simulink library "cooperative"  (Simulink 7.4)
settings: Solver=ode45  SolverMode=SingleTasking  StartTime=0.0  StopTime=10.0  RelTol=1e-3
undefined symbols (not defined in the file): ATRFunctions, g_AssignmentAlgorithm, g_CommandTurnRadius, g_CoordinationDelayDen, g_DefaultWaypointAltitude, g_EntityTypes, g_MaxNumberTargets, g_MaxNumberVehicles, g_MaxReassignmentDeltaTime, g_ObjectMessageIDs, g_OptionSaveDataAVDS, g_SampleTime, g_SensorRollLimitDeg, g_TargetStates, g_Tasks, g_TruthMemory, g_TypeAssignment, g_VehicleInputFiles, g_VehicleMemory, g_VehicleTypes, g_WaypointDefinitions, g_WaypointTypes
libraries: cooperative x23
(part 3 of 3)

== system cooperative/UAV1/ReceiveTruth/ImplementNewAssignment/VehicleAlive ==
  In1 : Inport
  In2 : Inport  Port=2
  Enable : EnablePort
  Bus Selector1 : BusSelector  OutputSignals=ChangeAssignmentFlagSelf
  Greater : Subsystem
  NewAssignment : Subsystem  TreatAsAtomicUnit=on
  Selector : Selector  InputPortWidth=g_MaxNumberVehicles  IndexOptions=Index vector (port)  Indices=[1 3]  OutputSizes=1
  wires:
  Bus Selector1/1 -> Selector/1  "<ChangeAssignmentFlagSelf>"
  Selector/1 -> Greater/1(Signal)
  In1/1 -> NewAssignment/1(VehicleID), Selector/2
  Greater/1(Greater?) -> NewAssignment/Enable
  In2/1 -> Bus Selector1/1

== system cooperative/UAV1/SendMessages/SendATRTime/Enabled Subsystem ==
  ATRTime : Inport
  Enable : EnablePort
  Digital Clock : DigitalClock  SampleTime=g_SampleTime
  SaveWaypointIndex : DataStoreWrite  DataStoreName=ATRTime  SampleTime=g_SampleTime
  TimeStamp : Outport
  wires:
  ATRTime/1 -> SaveWaypointIndex/1
  Digital Clock/1 -> TimeStamp/1

== system cooperative/UAV1/SendMessages/SendAuctionData/Enabled Subsystem ==
  MessageNumber : Inport
  Enable : EnablePort
  Data Store Write : DataStoreWrite  DataStoreName=LastMessageNumber  SampleTime=g_SampleTime
  Digital Clock : DigitalClock  SampleTime=g_SampleTime
  TimeStamp : Outport
  wires:
  MessageNumber/1 -> Data Store Write/1
  Digital Clock/1 -> TimeStamp/1

== system cooperative/UAV1/SendMessages/SendChangedStatus/Enabled Subsystem ==
  Enable : EnablePort
  Digital Clock : DigitalClock  SampleTime=g_SampleTime
  TimeStamp : Outport
  wires:
  Digital Clock/1 -> TimeStamp/1

== system cooperative/UAV1/SendMessages/SendPositionFlag/Enabled Subsystem ==
  PositionFlag : Inport
  Enable : EnablePort
  Digital Clock : DigitalClock  SampleTime=g_SampleTime
  SaveWaypointIndex : DataStoreWrite  DataStoreName=PositionFlag  SampleTime=g_SampleTime
  TimeStamp : Outport
  wires:
  Digital Clock/1 -> TimeStamp/1
  PositionFlag/1 -> SaveWaypointIndex/1

== system cooperative/UAV1/SendMessages/SendPositionID/Enabled Subsystem ==
  PositionSendFlag Time : Inport
  Enable : EnablePort
  Data Store Write : DataStoreWrite  DataStoreName=PositionsSendFlagTime  SampleTime=g_SampleTime
  Digital Clock : DigitalClock  SampleTime=g_SampleTime
  TimeStamp : Outport
  wires:
  PositionSendFlag Time/1 -> Data Store Write/1
  Digital Clock/1 -> TimeStamp/1

== system cooperative/UAV1/SendMessages/SendTargetAttacked/Enabled Subsystem ==
  "TargetAttacked " : Inport
  Enable : EnablePort
  Digital Clock : DigitalClock  SampleTime=g_SampleTime
  SaveWaypointIndex : DataStoreWrite  DataStoreName=TargetAttacked  SampleTime=g_SampleTime
  TimeStamp : Outport
  wires:
  Digital Clock/1 -> TimeStamp/1
  "TargetAttacked "/1 -> SaveWaypointIndex/1

== system cooperative/UAV1/SendMessages/SendTargetStatus/Enabled Subsystem ==
  Enable : EnablePort
  Digital Clock : DigitalClock  SampleTime=g_SampleTime
  TimeStamp : Outport
  wires:
  Digital Clock/1 -> TimeStamp/1

== system cooperative/UAV1/SendMessages/SendTaskBenefits/Enabled Subsystem ==
  ReplanRound : Inport
  Enable : EnablePort
  Data Store Write : DataStoreWrite  DataStoreName=LastReplanRound  SampleTime=g_SampleTime
  Digital Clock : DigitalClock  SampleTime=g_SampleTime
  TimeStamp : Outport
  wires:
  ReplanRound/1 -> Data Store Write/1
  Digital Clock/1 -> TimeStamp/1

== system cooperative/UAV1/SendMessages/SendTriggerReplan/Enabled Subsystem ==
  Enable : EnablePort
  Digital Clock : DigitalClock  SampleTime=g_SampleTime
  TimeStamp : Outport
  wires:
  Digital Clock/1 -> TimeStamp/1

== system cooperative/UAV1/SendMessages/SendWaypointNumber/Enabled Subsystem ==
  Waypoint : Inport
  Enable : EnablePort
  Digital Clock : DigitalClock  SampleTime=g_SampleTime
  SaveWaypointIndex : DataStoreWrite  DataStoreName=WaypoinNumber  SampleTime=g_SampleTime
  TimeStamp : Outport
  wires:
  Digital Clock/1 -> TimeStamp/1
  Waypoint/1 -> SaveWaypointIndex/1

== system cooperative/UAV1/SendTruth/SendNewAssignment/Changed1 ==
  Signal : Inport
  Relational Operator3 : RelationalOperator  Operator=>  InputSameDT=on
  Unit Delay : UnitDelay  SampleTime=g_SampleTime
  Greater? : Outport
  wires:
  Unit Delay/1 -> Relational Operator3/2
  Relational Operator3/1 -> Greater?/1
  Signal/1 -> Relational Operator3/1, Unit Delay/1

== system cooperative/UAV1/SendTruth/SendNewAssignment/Enabled Subsystem ==
  Enable : EnablePort
  Digital Clock : DigitalClock  SampleTime=g_SampleTime
  TimeStamp : Outport
  wires:
  Digital Clock/1 -> TimeStamp/1

== system cooperative/UAV1/SendTruth/SendTargetStatus/Enabled Subsystem ==
  TargetStatus : Inport
  Enable : EnablePort
  Data Store Write : DataStoreWrite  DataStoreName=TargetStatus  SampleTime=g_SampleTime
  Digital Clock : DigitalClock  SampleTime=g_SampleTime
  TimeStamp : Outport
  wires:
  Digital Clock/1 -> TimeStamp/1
  TargetStatus/1 -> Data Store Write/1

== system cooperative/UAV1/SendTruth/SendTrackList/Enabled Subsystem ==
  TrackList : Inport
  Enable : EnablePort
  Data Store Write : DataStoreWrite  DataStoreName=TrackList  SampleTime=g_SampleTime
  Digital Clock : DigitalClock  SampleTime=g_SampleTime
  TimeStamp : Outport
  wires:
  Digital Clock/1 -> TimeStamp/1
  TrackList/1 -> Data Store Write/1

== system cooperative/UAV1/SendTruth/SendVehicleIsDead/Enabled Subsystem ==
  State : Inport
  Enable : EnablePort
  Digital Clock : DigitalClock  SampleTime=g_SampleTime
  Save : DataStoreWrite  DataStoreName=VehicleIDead  SampleTime=g_SampleTime
  TimeStamp : Outport
  wires:
  Digital Clock/1 -> TimeStamp/1
  State/1 -> Save/1

== system cooperative/UAV1/SendTruth/SendWeaponsRelease/Enabled Subsystem ==
  WeaponID : Inport
  Enable : EnablePort
  Data Store Write : DataStoreWrite  DataStoreName=WeaponID  SampleTime=g_SampleTime
  Digital Clock : DigitalClock  SampleTime=g_SampleTime
  TimeStamp : Outport
  wires:
  WeaponID/1 -> Data Store Write/1
  Digital Clock/1 -> TimeStamp/1

== system cooperative/UAV1/EmbeddedFlightSoftware/CooperationManager/Calculate Assignment/CapTransShip ==
  note: Calculate Assignment
      |
      | PURPOSE: Calculate the assignments for the vehicles based on the current
      |      state of the targets and vehicles.
      |
      | IMPLEMENTATION:
      | - CapTransShipIO - calculates the costs/bennefits associated with the vehicle
      |      task assignments. "CapTransShipIO" also formats the data into the input
      |      form expected by the assignment algorithm.
      | - Capacitative Transshipment Solver - this is an interface to a compiled S-function
      |      that implements a capacitated transhipment algorithm. It is used to select the
      |      target and task assignment for all of the vehicles.
      | - Assignment for Local Vehicle - uses the current vehicle's ID to select and output
      |      the target and task assignment for this vehicle.
  ComBusLocalIn : Inport  SampleTime=g_SampleTime
  ComBusIn : Inport  Port=2  SampleTime=g_SampleTime
  Enable : EnablePort
  Assignment for Local Vehicle : Subsystem
  Bus Selector1 : BusSelector  OutputSignals=VehicleID,EFS(com).TargetManager(com).Target Status.TargetStatus  OutputAsBus=on
  Bus Selector2 : BusSelector  OutputSignals=ETACostToSearch,TargetAttacked  OutputAsBus=on
  CapTransShipIOInS : S-Function  FunctionName=CapTransShipIOInS  Parameters=g_MaxNumberTargets,g_MaxNumberVehicles,g_Tasks.NumberTasks  EnableBusSupport=off
  Capacitative Transshipment Solver : S-Function  FunctionName=CapTranShipDll  Parameters=g_MaxNumberVehicles,g_MaxNumberTargets,g_Tasks.NumberTasks  EnableBusSupport=off
  Mux3 : Mux  Inputs=2
  Local Assignment : Outport  InitialOutput=[0,0,0]
  wires:
  Assignment for Local Vehicle/1(Out1) -> Local Assignment/1
  ComBusIn/1 -> Bus Selector2/1
  CapTransShipIOInS/1 -> Capacitative Transshipment Solver/1
  Mux3/1 -> CapTransShipIOInS/1
  Capacitative Transshipment Solver/1 -> Assignment for Local Vehicle/2(In2)  "Assignment"
  Bus Selector1/1 -> Mux3/1
  ComBusLocalIn/1 -> Bus Selector1/1, Assignment for Local Vehicle/1(In1)
  Bus Selector2/1 -> Mux3/2

== system cooperative/UAV1/EmbeddedFlightSoftware/CooperationManager/Calculate Assignment/DistAuctItCapTransShip ==
  ComBusLocalIn : Inport  SampleTime=g_SampleTime
  ComBusIn : Inport  Port=2  SampleTime=g_SampleTime
  SimBusIn : Inport  Port=3  SampleTime=g_SampleTime
  EnableType : Inport  Port=4  SampleTime=g_SampleTime
  Enable : EnablePort
  Assignment Algorithm : Subsystem
  Bus Creator : BusCreator  Inputs=2
  Message Processing : Subsystem
  Not Used : Constant  Value=[0 0]
  Replan Logic : Subsystem
  Store Benefits : Subsystem  TreatAsAtomicUnit=on
  Local Assignment : Outport
  AuctionData : Outport  Port=2
  wires:
  EnableType/1 -> Replan Logic/1(EnableType)
  Store Benefits/1(BenefitsStored) -> Assignment Algorithm/3(StoredBenefits)
  Assignment Algorithm/2(TargetStates) -> Store Benefits/3(TargetStates)
  Assignment Algorithm/3(StoreBenefits) -> Store Benefits/Enable
  Message Processing/1(NewBid) -> Assignment Algorithm/1(NewBid)
  Message Processing/2(NewAssignment) -> Assignment Algorithm/2(NewAssignment)
  Message Processing/3(RoundComplete) -> Assignment Algorithm/4(RoundComplete)
  Assignment Algorithm/1(AuctionData) -> AuctionData/1  "AuctionData"
  Replan Logic/1(ReplanTrigger) -> Assignment Algorithm/5(ReplanTrigger), Message Processing/4(ReplanTrigger)  "ReplanTrigger"
  ComBusLocalIn/1 -> Assignment Algorithm/6(CommBusLocalIn), Store Benefits/2(CommBusLocalIn), Message Processing/3(CommBusLocalIn)
  SimBusIn/1 -> Message Processing/2(SimBusIn)
  ComBusIn/1 -> Store Benefits/1(CommBusIn), Message Processing/1(CommBusIn)
  Not Used/1 -> Bus Creator/1
  Bus Creator/1 -> Local Assignment/1
  Assignment Algorithm/4(NewAssignmentTime) -> Bus Creator/2  "NewAssignmetTime"

== system cooperative/UAV1/EmbeddedFlightSoftware/CooperationManager/Calculate Assignment/DistItCapTransShip ==
  ComBusLocalIn : Inport  SampleTime=g_SampleTime
  ComBusIn : Inport  Port=2  SampleTime=g_SampleTime
  SimBusIn : Inport  Port=3  SampleTime=g_SampleTime
  EnableType : Inport  Port=4  SampleTime=g_SampleTime
  Enable : EnablePort
  Assignment Algorithm : Subsystem
  Bus Creator : BusCreator  Inputs=2
  Demux : Demux  Outputs=7  BusSelectionMode=on
  Iteration Logic : Subsystem
  Mux : Mux  Inputs=7
  Not Used : Constant  Value=[0 0]
  Replan Logic : Subsystem
  Send Benefits : Subsystem  TreatAsAtomicUnit=on
  Local Assignment : Outport  InitialOutput=[0,0,0]
  Algorithm Data : Outport  Port=2
  wires:
  EnableType/1 -> Replan Logic/1(EnableType)
  Assignment Algorithm/3(SendBenefitsTrigger) -> Send Benefits/Enable
  Assignment Algorithm/1(TargetStatesOut) -> Send Benefits/3(TargetStates)
  Assignment Algorithm/2(ReplanRoundOut) -> Send Benefits/4(ReplanRound)
  Replan Logic/1(ReplanTrigger) -> Assignment Algorithm/8(ReplanTrigger)
  Demux/7 -> Assignment Algorithm/7(Sync)
  Demux/6 -> Assignment Algorithm/6(SearchBenefits)
  Demux/5 -> Assignment Algorithm/5(TimeToComplete)
  Demux/4 -> Assignment Algorithm/4(TaskBenefits)
  Demux/3 -> Assignment Algorithm/3(TargetStatesIn)
  Demux/2 -> Assignment Algorithm/2(ReplanRoundIn)
  Demux/1 -> Assignment Algorithm/1(ActiveVehicles)
  Mux/1 -> Demux/1
  Iteration Logic/7(Sync) -> Mux/7
  Iteration Logic/6(SearchBenefits) -> Mux/6
  Iteration Logic/5(TimeToComplete) -> Mux/5
  Iteration Logic/4(TaskBenefits) -> Mux/4
  Iteration Logic/3(TargetStates) -> Mux/3
  Iteration Logic/2(ReplanRound) -> Mux/2
  Iteration Logic/1(ActiveVehicles) -> Mux/1
  ComBusLocalIn/1 -> Assignment Algorithm/9(CommBusLocalIn), Send Benefits/2(CommBusLocalIn)
  SimBusIn/1 -> Iteration Logic/2(SimBusIn)
  ComBusIn/1 -> Send Benefits/1(CommBusIn), Iteration Logic/1(CommBusIn)
  Send Benefits/1(Algorithm Data) -> Algorithm Data/1
  Not Used/1 -> Bus Creator/1  "Localassignment"
  Bus Creator/1 -> Local Assignment/1
  Assignment Algorithm/4(NewAssignmentTime) -> Bus Creator/2  "NewAssignmentTime"

== system cooperative/UAV1/EmbeddedFlightSoftware/CooperationManager/Calculate Assignment/ItCapTransShip ==
  note: ItCapTransShip
      |
      | PURPOSE: .
      |
      | IMPLEMENTATION:
      | - .
      | - .
      | - .
  ComBusLocalIn : Inport  SampleTime=g_SampleTime
  ComBusIn : Inport  Port=2  SampleTime=g_SampleTime
  SimBusIn : Inport  Port=3  SampleTime=g_SampleTime
  Enable : EnablePort
  Bus Selector : BusSelector  OutputSignals=PositionID,WaypointIndex,TriggerReplan  OutputAsBus=on
  Bus Selector1 : BusSelector  OutputSignals=VehicleID,EFS(com).TargetManager(com).SensedTargetInformation.Targets,EFS(com).TargetManager(com).Target Status.TargetStatus,EFS(com).SensorManager(com).ATR Combined.Desired Headings.DesiredHeadings01,EFS(com).SensorManager(com).ATR Combined.Desired Headings.DesiredHeadings02,EFS(com).SensorManager(com).ATR Combined.Desired Headings.DesiredHeadings03,EFS(com).SensorManager(com).ATR Combined.Desired Headings.DesiredHeadings04,Dynamics(com).TacticalManuevering.CommandTurnRadius,Dynamics(com).TacticalManuevering.WayPointNumber,Dynamics(com).TacticalManuevering.WayPointTypeCurrent  OutputAsBus=on
  Bus Selector2 : BusSelector  OutputSignals=ExternalTruth.VehicleIsDead  OutputAsBus=on
  MultiTaskAssignIOS : S-Function  FunctionName=MultiTaskAssignIOS  Parameters=g_TypeAssignment.ItCapTransShip,g_MaxNumberTargets,g_MaxNumberVehicles  EnableBusSupport=off
  Mux : Mux  Inputs=3
  Local Assignment : Outport  InitialOutput=[0,0,0]
  wires:
  Bus Selector2/1 -> Mux/2
  SimBusIn/1 -> Bus Selector2/1
  Mux/1 -> MultiTaskAssignIOS/1
  Bus Selector1/1 -> Mux/3
  Bus Selector/1 -> Mux/1
  MultiTaskAssignIOS/1 -> Local Assignment/1
  ComBusIn/1 -> Bus Selector/1
  ComBusLocalIn/1 -> Bus Selector1/1

== system cooperative/UAV1/EmbeddedFlightSoftware/CooperationManager/Calculate Assignment/ItJacobi ==
  note: ItCapTransShip
      |
      | PURPOSE: .
      |
      | IMPLEMENTATION:
      | - .
      | - .
      | - .
  ComBusLocalIn : Inport  SampleTime=g_SampleTime
  ComBusIn : Inport  Port=2  SampleTime=g_SampleTime
  SimBusIn : Inport  Port=3  SampleTime=g_SampleTime
  Enable : EnablePort
  Bus Selector : BusSelector  OutputSignals=PositionID,WaypointIndex,TriggerReplan  OutputAsBus=on
  Bus Selector1 : BusSelector  OutputSignals=VehicleID,EFS(com).TargetManager(com).SensedTargetInformation.Targets,EFS(com).TargetManager(com).Target Status.TargetStatus,EFS(com).SensorManager(com).ATR Combined.Desired Headings.DesiredHeadings01,EFS(com).SensorManager(com).ATR Combined.Desired Headings.DesiredHeadings02,EFS(com).SensorManager(com).ATR Combined.Desired Headings.DesiredHeadings03,EFS(com).SensorManager(com).ATR Combined.Desired Headings.DesiredHeadings04,Dynamics(com).TacticalManuevering.CommandTurnRadius,Dynamics(com).TacticalManuevering.WayPointNumber,Dynamics(com).TacticalManuevering.WayPointTypeCurrent  OutputAsBus=on
  Bus Selector3 : BusSelector  OutputSignals=ExternalTruth.VehicleIsDead  OutputAsBus=on
  MultiTaskAssignIOS : S-Function  FunctionName=MultiTaskAssignIOS  Parameters=g_TypeAssignment.ItAuctionJacobi,g_MaxNumberTargets,g_MaxNumberVehicles  EnableBusSupport=off
  Mux : Mux  Inputs=3
  Local Assignment : Outport  InitialOutput=[0,0,0]
  wires:
  Bus Selector3/1 -> Mux/2
  SimBusIn/1 -> Bus Selector3/1
  Mux/1 -> MultiTaskAssignIOS/1
  Bus Selector1/1 -> Mux/3
  Bus Selector/1 -> Mux/1
  MultiTaskAssignIOS/1 -> Local Assignment/1
  ComBusIn/1 -> Bus Selector/1
  ComBusLocalIn/1 -> Bus Selector1/1

== system cooperative/UAV1/EmbeddedFlightSoftware/CooperationManager/Calculate Assignment/MessageDisplay ==
  In1 : Inport
  Enable : EnablePort
  MessageDisplayS : S-Function  Priority=1  FunctionName=MessageDisplayS  Parameters='Replan'  EnableBusSupport=off
  wires:
  In1/1 -> MessageDisplayS/1

== system cooperative/UAV1/EmbeddedFlightSoftware/CooperationManager/Calculate Assignment/Relative Bennifits ==
  note: ItCapTransShip
      |
      | PURPOSE: .
      |
      | IMPLEMENTATION:
      | - .
      | - .
      | - .
  ComBusLocalIn : Inport  SampleTime=g_SampleTime
  ComBusIn : Inport  Port=2  SampleTime=g_SampleTime
  SimBusIn : Inport  Port=3  SampleTime=g_SampleTime
  Enable : EnablePort
  Bus Selector1 : BusSelector  OutputSignals=VehicleID,EFS(com).TargetManager(com).SensedTargetInformation.Targets,EFS(com).TargetManager(com).Target Status.TargetStatus,EFS(com).SensorManager(com).ATR Combined.Desired Headings.DesiredHeadings01,EFS(com).SensorManager(com).ATR Combined.Desired Headings.DesiredHeadings02,EFS(com).SensorManager(com).ATR Combined.Desired Headings.DesiredHeadings03,EFS(com).SensorManager(com).ATR Combined.Desired Headings.DesiredHeadings04,Dynamics(com).TacticalManuevering.CommandTurnRadius,Dynamics(com).TacticalManuevering.WayPointNumber,Dynamics(com).TacticalManuevering.WayPointTypeCurrent  OutputAsBus=on
  Bus Selector3 : BusSelector  OutputSignals=PositionID,WaypointIndex,TriggerReplan  OutputAsBus=on
  Bus Selector4 : BusSelector  OutputSignals=ExternalTruth.VehicleIsDead  OutputAsBus=on
  MultiTaskAssignIOS : S-Function  FunctionName=MultiTaskAssignIOS  Parameters=g_TypeAssignment.RelativeBenefits,g_MaxNumberTargets,g_MaxNumberVehicles  EnableBusSupport=off
  Mux : Mux  Inputs=3
  Local Assignment : Outport  InitialOutput=[0,0,0]
  wires:
  Bus Selector4/1 -> Mux/2
  SimBusIn/1 -> Bus Selector4/1
  Mux/1 -> MultiTaskAssignIOS/1
  Bus Selector1/1 -> Mux/3
  Bus Selector3/1 -> Mux/1
  MultiTaskAssignIOS/1 -> Local Assignment/1
  ComBusIn/1 -> Bus Selector3/1
  ComBusLocalIn/1 -> Bus Selector1/1

== system cooperative/UAV1/EmbeddedFlightSoftware/CooperationManager/Enable Reassignment/Assignment Time Delay ==
  note: Coordination Timing
      |
      | PURPOSE: This is a time delay to make sure that all of the
      |  other vehicle have had time to calculate the new
      |  routes. If they still have not the replan algorithm will
      |  not use that vehicle's old information.
  In : Inport  SampleTime=g_SampleTime
  Discrete Transfer Fcn : DiscreteTransferFcn  Denominator=g_CoordinationDelayDen  SampleTime=g_SampleTime
  InDelayed : Outport
  wires:
  Discrete Transfer Fcn/1 -> InDelayed/1
  In/1 -> Discrete Transfer Fcn/1

== system cooperative/UAV1/EmbeddedFlightSoftware/CooperationManager/Enable Reassignment/Changed ==
  Signal : Inport
  Relational Operator3 : RelationalOperator  Operator=~=  InputSameDT=on
  Unit Delay : UnitDelay  SampleTime=g_SampleTime
  Increased? : Outport
  wires:
  Unit Delay/1 -> Relational Operator3/2
  Relational Operator3/1 -> Increased?/1
  Signal/1 -> Relational Operator3/1, Unit Delay/1

== system cooperative/UAV1/EmbeddedFlightSoftware/CooperationManager/Enable Reassignment/Changed1 ==
  Signal : Inport
  Relational Operator3 : RelationalOperator  Operator=~=  InputSameDT=on
  Unit Delay : UnitDelay  SampleTime=g_SampleTime
  Changed? : Outport
  wires:
  Unit Delay/1 -> Relational Operator3/2
  Relational Operator3/1 -> Changed?/1
  Signal/1 -> Relational Operator3/1, Unit Delay/1

== system cooperative/UAV1/EmbeddedFlightSoftware/CooperationManager/Enable Reassignment/Changed2 ==
  Signal : Inport
  Relational Operator3 : RelationalOperator  Operator=~=  InputSameDT=on
  Unit Delay : UnitDelay  SampleTime=g_SampleTime
  Changed? : Outport
  wires:
  Signal/1 -> Unit Delay/1, Relational Operator3/1
  Relational Operator3/1 -> Changed?/1
  Unit Delay/1 -> Relational Operator3/2

== system cooperative/UAV1/EmbeddedFlightSoftware/CooperationManager/Task List/Update Task List ==
  note: Task List
  Vehicle ID : Inport  SampleTime=g_SampleTime
  TargetStatus : Inport  Port=2  SampleTime=g_SampleTime
  Enable : EnablePort
  Mux : Mux  Inputs=2
  TargetStatusS : S-Function  FunctionName=TaskListS  Parameters=g_MaxNumberTargets  EnableBusSupport=off
  "Write Last Target Status " : DataStoreWrite  DataStoreName=LastTargetStatus  SampleTime=g_SampleTime
  UnassignedTaskFlag : Outport
  wires:
  TargetStatusS/1 -> UnassignedTaskFlag/1
  Mux/1 -> TargetStatusS/1
  Vehicle ID/1 -> Mux/1
  TargetStatus/1 -> Mux/2, "Write Last Target Status "/1

== system cooperative/UAV1/EmbeddedFlightSoftware/RouteManager/ReplanSingle/Replan ==
  note: RouteSelection
      |
      | PURPOSE: Calculates the ETA, cost and waypoint trajectory for the lowest
      |      cost flyable path to each of the targets, to accomplish the appropriate task,
      |      and stores the data for later use.
      |
      | Implementation:
      | - ReplanRoutes- calls the function, "ReplanRoutes" to do the calculations. The
      |      lowest cost set of waypoints for each known target is stored in the appropriate
      |      location in the global structure "VehicleMemory.RouteManager".
  In1 : Inport
  Enable : EnablePort
  Bus Creator : BusCreator
  Bus Selector : BusSelector  OutputSignals=Local Bus.VehicleID,Vehicle (Sim).EFS(sim).RouteManager(sim).VehicleFinished.Vehicle Finished,Local Bus.Dynamics(com).TacticalManuevering.CommandTurnRadius,Local Bus.Dynamics(com).AC Dynamics.Position_x,Local Bus.Dynamics(com).AC Dynamics.Position_y,Local Bus.Dynamics(com).AC Dynamics.Altitude,Local Bus.Dynamics(com).AC Dynamics.Psi,Local Bus.Dynamics(com).AC Dynamics.V North,Local Bus.Dynamics(com).AC Dynamics.V East,Local Bus.Dynamics(com).TacticalManuevering.CommandVelocity,Local Bus.Dynamics(com).TacticalManuevering.WayPointNumber,Local Bus.EFS(com).RouteManager(com).TaskStatus.Task Finished,Local Bus.EFS(com).TargetManager(com).Target Status.TargetStatus,Local Bus.EFS(com).SensorManager(com).ATR Combined.Desired Headings,TargetState  OutputAsBus=on
  Demux : Demux  Outputs=[g_MaxNumberTargets,g_MaxNumberTargets,g_MaxNumberTargets]
  Digital Clock : DigitalClock  SampleTime=g_SampleTime
  ReplanRoutes : S-Function  FunctionName=ReplanRoutesS  Parameters=g_MaxNumberTargets  EnableBusSupport=off
  ReplanETAsCosts : Outport
  wires:
  Demux/2 -> Bus Creator/3  "TargetETAs"
  Digital Clock/1 -> Bus Creator/1  "ReplanTime"
  In1/1 -> Bus Selector/1
  Bus Selector/1 -> ReplanRoutes/1
  Demux/3 -> Bus Creator/4  "TargetToSearchDist"
  Bus Creator/1 -> ReplanETAsCosts/1  "Replan ETAs and Costs"
  ReplanRoutes/1 -> Demux/1
  Demux/1 -> Bus Creator/2  "TargetCosts"

== system cooperative/UAV1/EmbeddedFlightSoftware/RouteManager/ReplanSingle/RouteSelection ==
  note: RouteSelection
      |
      | PURPOSE: This manager implements waypoints for the route selected for this
      | vehicle during the vehicle/target assignment in the cooperation manager.
      |
      | Implementation:
      | - RouteSelection - calls the function "RouteSelection" to implement waypoints
      |      for the route selected.
  In1 : Inport
  Enable : EnablePort
  RouteSelection : S-Function  FunctionName=RouteSelectionS  EnableBusSupport=off
  wires:
  In1/1 -> RouteSelection/1

== system cooperative/UAV1/EmbeddedFlightSoftware/RouteManager/Task Status/Alive Time ==
  Local (Comm) : Inport  SampleTime=g_SampleTime
  Enable : EnablePort
  Bus Selector4 : BusSelector  OutputSignals=VehicleID
  Digital Clock : DigitalClock  SampleTime=g_SampleTime
  Mux : Mux  Inputs=2
  S-Function : S-Function  FunctionName=MonteCarloMetricS  Parameters='AliveTimeSeconds'  EnableBusSupport=off
  wires:
  Bus Selector4/1 -> Mux/1  "<VehicleID>"
  Local (Comm)/1 -> Bus Selector4/1
  Mux/1 -> S-Function/1
  Digital Clock/1 -> Mux/2

== system cooperative/UAV1/EmbeddedFlightSoftware/RouteManager/Task Status/D Latch ==
  Enable : Inport
  In : Inport  Port=2  SampleTime=g_SampleTime
  D Latch : Subsystem  TreatAsAtomicUnit=on
  Latched : Outport  InitialOutput=0
  wires:
  Enable/1 -> D Latch/Enable
  D Latch/1(Q) -> Latched/1
  In/1 -> D Latch/1(D)

== system cooperative/UAV1/EmbeddedFlightSoftware/RouteManager/Task Status/D Latch1 ==
  Enable : Inport
  In : Inport  Port=2  SampleTime=g_SampleTime
  D Latch : Subsystem  TreatAsAtomicUnit=on
  Latched : Outport  InitialOutput=0
  wires:
  In/1 -> D Latch/1(D)
  D Latch/1(Q) -> Latched/1
  Enable/1 -> D Latch/Enable

== system cooperative/UAV1/EmbeddedFlightSoftware/RouteManager/Task Status/D Latch2 ==
  Enable : Inport
  In : Inport  Port=2  SampleTime=g_SampleTime
  D Latch : Subsystem  TreatAsAtomicUnit=on
  Latched : Outport  InitialOutput=0
  wires:
  Enable/1 -> D Latch/Enable
  D Latch/1(Q) -> Latched/1
  In/1 -> D Latch/1(D)

== system cooperative/UAV1/EmbeddedFlightSoftware/RouteManager/Task Status/Task Failed Check ==
  Local (Comm) : Inport
  Bus Selector1 : BusSelector  OutputSignals=Dynamics(com).TacticalManuevering.WayPointTypeCurrent,EFS(com).TargetManager(com).Target Status.TargetStatus
  Create Last Task : DataStoreMemory  DataStoreName=LastWaypointType
  Create Last Task1 : DataStoreMemory  DataStoreName=LastTargetState  InitialValue=g_TargetStates.StateUndefined*ones(g_MaxNumberTargets,1)
  Logical Operator : Logic  Operator=OR
  Read Last Task : DataStoreRead  DataStoreName=LastWaypointType  SampleTime=g_SampleTime
  Read Last Task1 : DataStoreRead  DataStoreName=LastTargetState  SampleTime=g_SampleTime
  Relational Operator1 : RelationalOperator  Operator=~=  InputSameDT=on
  Relational Operator4 : RelationalOperator  Operator=~=  InputSameDT=on
  Task Failed Check : Subsystem  TreatAsAtomicUnit=on
  TaskFailed : Outport
  wires:
  Relational Operator1/1 -> Logical Operator/2
  Read Last Task1/1 -> Task Failed Check/2(LastTargetState), Relational Operator1/2
  Bus Selector1/2 -> Relational Operator1/1  "<TargetStatus>"
  Relational Operator4/1 -> Logical Operator/1
  Logical Operator/1 -> Task Failed Check/Enable
  Task Failed Check/1(TaskFailed) -> TaskFailed/1
  Bus Selector1/1 -> Relational Operator4/2  "<WayPointTypeCurrent>"
  Read Last Task/1 -> Relational Operator4/1
  Local (Comm)/1 -> Task Failed Check/1(Local (Comm)), Bus Selector1/1

== system cooperative/UAV1/EmbeddedFlightSoftware/RouteManager/Task Status/VehicleType ==
  VehicleID : Inport
  Enable : EnablePort
  EntityType : MATLABFcn  MATLABFcn=g_VehicleTypes(g_VehicleMemory(u).VehicleType).EntityType
  Relational Operator4 : RelationalOperator  Operator=~=  InputSameDT=on
  WaypointTypes.EndTask1 : Constant  Value=g_EntityTypes.Munition
  NotMunition : Outport  InitialOutput=0
  wires:
  WaypointTypes.EndTask1/1 -> Relational Operator4/2
  EntityType/1 -> Relational Operator4/1  "TaskCompleted"
  VehicleID/1 -> EntityType/1
  Relational Operator4/1 -> NotMunition/1  "NotMunition"

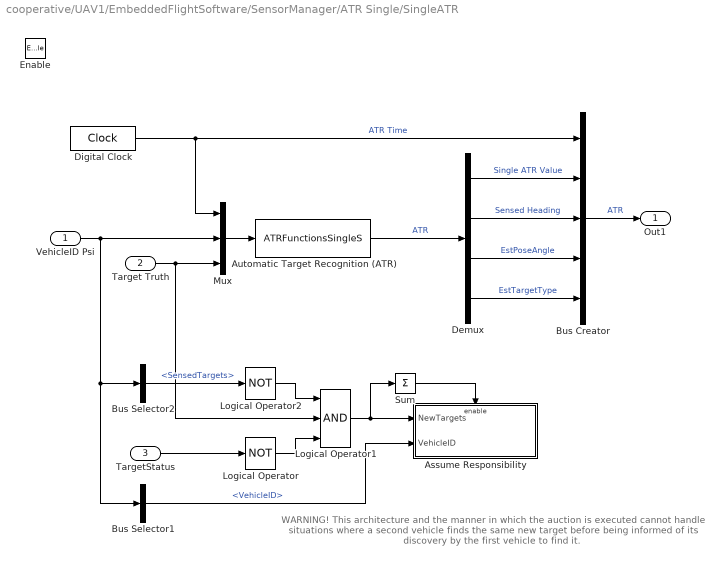
== system cooperative/UAV1/EmbeddedFlightSoftware/SensorManager/ATR Single/SingleATR ==
  note: WARNING!
      | This architecture and the manner in which
      | the auction is executed cannot handle
      | situations where a second vehicle finds the
      | same new target before being informed of its
      | discovery by the first vehicle to find it.
  VehicleID Psi : Inport
  "Target Truth " : Inport  Port=2
  TargetStatus : Inport  Port=3  SampleTime=g_SampleTime
  Enable : EnablePort
  Assume Responsibility : Subsystem  TreatAsAtomicUnit=on
  Automatic Target Recognition (ATR) : S-Function  FunctionName=ATRFunctionsSingleS  Parameters=g_MaxNumberTargets  EnableBusSupport=off
  Bus Creator : BusCreator  Inputs=5
  Bus Selector1 : BusSelector  OutputSignals=VehicleID
  Bus Selector2 : BusSelector  OutputSignals=SensedTargets
  Demux : Demux  Outputs=[g_MaxNumberTargets,g_MaxNumberTargets,g_MaxNumberTargets,g_MaxNumberTargets]
  Digital Clock : DigitalClock  SampleTime=g_SampleTime
  Logical Operator : Logic  Operator=NOT  Inputs=1
  Logical Operator1 : Logic  Inputs=3
  Logical Operator2 : Logic  Operator=NOT  Inputs=1
  Mux : Mux  Inputs=3
  Sum : Sum  Inputs=+  SaturateOnIntegerOverflow=on  InputSameDT=on  OutDataTypeStr=Inherit: Same as first input
  Out1 : Outport
  wires:
  Logical Operator2/1 -> Logical Operator1/1
  Bus Selector2/1 -> Logical Operator2/1  "<SensedTargets>"
  TargetStatus/1 -> Logical Operator/1
  Sum/1 -> Assume Responsibility/Enable
  Bus Selector1/1 -> Assume Responsibility/2(VehicleID)  "<VehicleID>"
  Logical Operator1/1 -> Assume Responsibility/1(NewTargets), Sum/1
  Logical Operator/1 -> Logical Operator1/3
  Demux/4 -> Bus Creator/5  "EstTargetType"
  Automatic Target Recognition (ATR)/1 -> Demux/1  "ATR"
  Demux/3 -> Bus Creator/4  "EstPoseAngle"
  Demux/2 -> Bus Creator/3  "Sensed Heading"
  "Target Truth "/1 -> Logical Operator1/2, Mux/3
  Bus Creator/1 -> Out1/1  "ATR"
  VehicleID Psi/1 -> Bus Selector2/1, Bus Selector1/1, Mux/2
  Mux/1 -> Automatic Target Recognition (ATR)/1
  Demux/1 -> Bus Creator/2  "Single ATR Value"
  Digital Clock/1 -> Mux/1, Bus Creator/1  "ATR Time"

== system cooperative/UAV1/ReceiveTruth/ImplementNewAssignment/VehicleAlive/Greater ==
  Signal : Inport
  Relational Operator3 : RelationalOperator  Operator=>  InputSameDT=on
  Unit Delay : UnitDelay  SampleTime=g_SampleTime
  Greater? : Outport
  wires:
  Unit Delay/1 -> Relational Operator3/2
  Relational Operator3/1 -> Greater?/1
  Signal/1 -> Relational Operator3/1, Unit Delay/1

== system cooperative/UAV1/ReceiveTruth/ImplementNewAssignment/VehicleAlive/NewAssignment ==
  VehicleID : Inport
  Enable : EnablePort
  ImplementNewAssignment : S-Function  FunctionName=ImplementNewAssignmentS  EnableBusSupport=off
  wires:
  VehicleID/1 -> ImplementNewAssignment/1

== system cooperative/UAV1/EmbeddedFlightSoftware/CooperationManager/Calculate Assignment/CapTransShip/Assignment for Local Vehicle ==
  note: Assignment for Local Vehicle
      |
      | PURPOSE: Output the target and task assignment
      |      for the local vehicle..
      |
      | IMPLEMENTATION: This block uses a"Selector" Block to select the target and task assignment
      |       based on the VehicleID signal.
  note: Note: new assignment is implemented in the route manager.
  In1 : Inport  SampleTime=g_SampleTime
  In2 : Inport  Port=2  SampleTime=g_SampleTime
  Bus Creator : BusCreator  Inputs=3
  Bus Selector : BusSelector  OutputSignals=VehicleID
  Constant : Constant  Value=0
  Demux : Demux  Outputs=2
  SelectedSignals : MATLABFcn  MATLABFcn=[u(1),g_MaxNumberVehicles+u(1)]
  Selector : Selector  InputPortWidth=2*g_MaxNumberVehicles + 1  IndexOptions=Index vector (port)  Indices=[1 3]  OutputSizes=1
  Out1 : Outport
  wires:
  In1/1 -> Bus Selector/1
  Bus Creator/1 -> Out1/1  "Assignment - Local"
  Demux/1 -> Bus Creator/1  "Target Assignment - Local"
  Demux/2 -> Bus Creator/2  "Task Assignment  - Local"
  Bus Selector/1 -> SelectedSignals/1  "<VehicleID>"
  In2/1 -> Selector/1
  Constant/1 -> Bus Creator/3  "NewAssignmentFlag"
  SelectedSignals/1 -> Selector/2
  Selector/1 -> Demux/1

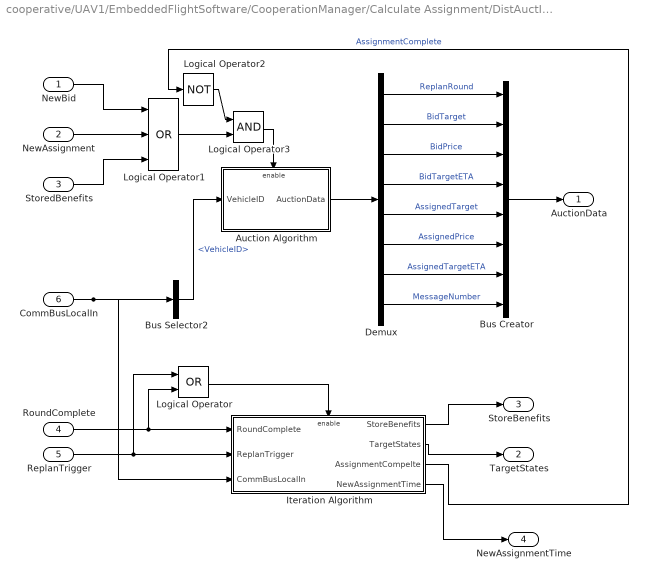
== system cooperative/UAV1/EmbeddedFlightSoftware/CooperationManager/Calculate Assignment/DistAuctItCapTransShip/Assignment Algorithm ==
  NewBid : Inport
  NewAssignment : Inport  Port=2
  StoredBenefits : Inport  Port=3
  RoundComplete : Inport  Port=4
  ReplanTrigger : Inport  Port=5
  CommBusLocalIn : Inport  Port=6
  Auction Algorithm : Subsystem  TreatAsAtomicUnit=on
  Bus Creator : BusCreator  Inputs=8
  Bus Selector2 : BusSelector  OutputSignals=VehicleID
  Demux : Demux  Outputs=[2, g_MaxNumberVehicles,g_MaxNumberVehicles,g_MaxNumberVehicles,g_MaxNumberVehicles,g_MaxNumberVehicles,g_MaxNumberVehicles,1]
  Iteration Algorithm : Subsystem  TreatAsAtomicUnit=on
  Logical Operator : Logic  Operator=OR
  Logical Operator1 : Logic  Operator=OR  Inputs=3
  Logical Operator2 : Logic  Operator=NOT  Inputs=21
  Logical Operator3 : Logic
  AuctionData : Outport
  TargetStates : Outport  Port=2
  StoreBenefits : Outport  Port=3
  NewAssignmentTime : Outport  Port=4
  wires:
  Logical Operator3/1 -> Auction Algorithm/Enable
  Logical Operator2/1 -> Logical Operator3/1
  Logical Operator1/1 -> Logical Operator3/2
  Iteration Algorithm/3(AssignmentCompelte) -> Logical Operator2/1  "AssignmentComplete"
  StoredBenefits/1 -> Logical Operator1/3
  Demux/3 -> Bus Creator/3  "BidPrice"
  Bus Selector2/1 -> Auction Algorithm/1(VehicleID)  "<VehicleID>"
  CommBusLocalIn/1 -> Iteration Algorithm/3(CommBusLocalIn), Bus Selector2/1
  NewBid/1 -> Logical Operator1/1
  NewAssignment/1 -> Logical Operator1/2
  Auction Algorithm/1(AuctionData) -> Demux/1
  Demux/6 -> Bus Creator/6  "AssignedPrice"
  Logical Operator/1 -> Iteration Algorithm/Enable
  RoundComplete/1 -> Logical Operator/2, Iteration Algorithm/1(RoundComplete)
  ReplanTrigger/1 -> Logical Operator/1, Iteration Algorithm/2(ReplanTrigger)
  Iteration Algorithm/2(TargetStates) -> TargetStates/1
  Iteration Algorithm/1(StoreBenefits) -> StoreBenefits/1
  Bus Creator/1 -> AuctionData/1
  Demux/8 -> Bus Creator/8  "MessageNumber"
  Demux/5 -> Bus Creator/5  "AssignedTarget"
  Demux/4 -> Bus Creator/4  "BidTargetETA"
  Demux/2 -> Bus Creator/2  "BidTarget"
  Demux/1 -> Bus Creator/1  "ReplanRound"
  Demux/7 -> Bus Creator/7  "AssignedTargetETA"
  Iteration Algorithm/4(NewAssignmentTime) -> NewAssignmentTime/1

== system cooperative/UAV1/EmbeddedFlightSoftware/CooperationManager/Calculate Assignment/DistAuctItCapTransShip/Message Processing ==
  CommBusIn : Inport
  SimBusIn : Inport  Port=2
  CommBusLocalIn : Inport  Port=3
  ReplanTrigger : Inport  Port=4
  Bus Selector1 : BusSelector  OutputSignals=AuctionData
  Bus Selector2 : BusSelector  OutputSignals=VehicleID
  Bus Selector4 : BusSelector  OutputSignals=ExternalTruth.VehicleIsDead  OutputAsBus=on
  Demux : Demux  Outputs=[1 1 1]
  Logical Operator : Logic  Operator=NOT
  Mux1 : Mux
  S-Function : S-Function  FunctionName=DAINF_MessageControlS  EnableBusSupport=off
  NewBid : Outport
  NewAssignment : Outport  Port=2
  RoundComplete : Outport  Port=3
  wires:
  Demux/3 -> RoundComplete/1
  Demux/2 -> NewAssignment/1
  Demux/1 -> NewBid/1
  S-Function/1 -> Demux/1
  Mux1/1 -> S-Function/1
  Bus Selector2/1 -> Mux1/1  "<VehicleID>"
  CommBusLocalIn/1 -> Bus Selector2/1
  Logical Operator/1 -> Mux1/2  "ActiveVehicles"
  ReplanTrigger/1 -> Mux1/4  "ReplanTrigger"
  Bus Selector1/1 -> Mux1/3  "<AuctionData>"
  CommBusIn/1 -> Bus Selector1/1
  Bus Selector4/1 -> Logical Operator/1
  SimBusIn/1 -> Bus Selector4/1

== system cooperative/UAV1/EmbeddedFlightSoftware/CooperationManager/Calculate Assignment/DistAuctItCapTransShip/Replan Logic ==
  EnableType : Inport
  Constant : Constant
  Constant1 : Constant
  Constant2 : Constant  Value=0
  Multiport Switch : MultiPortSwitch  Inputs=4  SaturateOnIntegerOverflow=on  InputSameDT=on
  Sum : Sum  Inputs=++|  SaturateOnIntegerOverflow=on  InputSameDT=on  OutDataTypeStr=Inherit: Same as first input
  ReplanTrigger : Outport
  wires:
  Constant1/1 -> Multiport Switch/5, Multiport Switch/3
  Constant2/1 -> Multiport Switch/4, Multiport Switch/2
  Multiport Switch/1 -> ReplanTrigger/1
  Sum/1 -> Multiport Switch/1
  Constant/1 -> Sum/1
  EnableType/1 -> Sum/2

== system cooperative/UAV1/EmbeddedFlightSoftware/CooperationManager/Calculate Assignment/DistAuctItCapTransShip/Store Benefits ==
  CommBusIn : Inport
  CommBusLocalIn : Inport  Port=2
  TargetStates : Inport  Port=3
  Enable : EnablePort  ShowOutputPort=on
  Demux : Demux  Outputs=[g_MaxNumberTargets,g_MaxNumberTargets,1]
  Mux : Mux  Inputs=5
  Mux1 : Mux  Inputs=10
  S-Function : S-Function  FunctionName=DINF_CalculateBenefitsS  Parameters=g_MaxNumberTargets,g_MaxNumberVehicles  EnableBusSupport=off
  S-Function1 : S-Function  FunctionName=DAINF_StoreBenefitsS  EnableBusSupport=off
  SimBusSelector : BusSelector  OutputSignals=Time,VehicleID,Dynamics(com).AC Dynamics.Position_x,Dynamics(com).AC Dynamics.Position_y,Dynamics(com).AC Dynamics.Psi,Dynamics(com).TacticalManuevering.WayPointNumber,EFS(com).TargetManager(com).SensedTargetInformation.Targets,EFS(com).SensorManager(com).ATR Combined.Desired Headings
  SimBusSelector1 : BusSelector  OutputSignals=VehicleID
  SimBusSelector2 : BusSelector  OutputSignals=TriggerReplan
  BenefitsStored : Outport  OutputWhenDisabled=reset  InitialOutput=[0]
  wires:
  SimBusSelector2/1 -> Mux1/10  "<TriggerReplan>"
  CommBusIn/1 -> SimBusSelector2/1
  Enable/1 -> BenefitsStored/1
  SimBusSelector1/1 -> Mux/1  "<VehicleID>"
  Mux/1 -> S-Function1/1
  TargetStates/1 -> Mux/5, Mux1/9  "TargetStates"
  SimBusSelector/6 -> Mux1/6  "<WayPointNumber>"
  SimBusSelector/8 -> Mux1/8  "<Desired Headings>"
  SimBusSelector/7 -> Mux1/7  "<Targets>"
  SimBusSelector/5 -> Mux1/5  "<Psi>"
  SimBusSelector/4 -> Mux1/4  "<Position_y>"
  SimBusSelector/3 -> Mux1/3  "<Position_x>"
  SimBusSelector/2 -> Mux1/2  "<VehicleID>"
  SimBusSelector/1 -> Mux1/1  "<Time>"
  CommBusLocalIn/1 -> SimBusSelector1/1, SimBusSelector/1
  Mux1/1 -> S-Function/1
  S-Function/1 -> Demux/1
  Demux/3 -> Mux/4  "SearchBenefit"
  Demux/2 -> Mux/3  "TimeToComplete"
  Demux/1 -> Mux/2  "TaskBenefits"

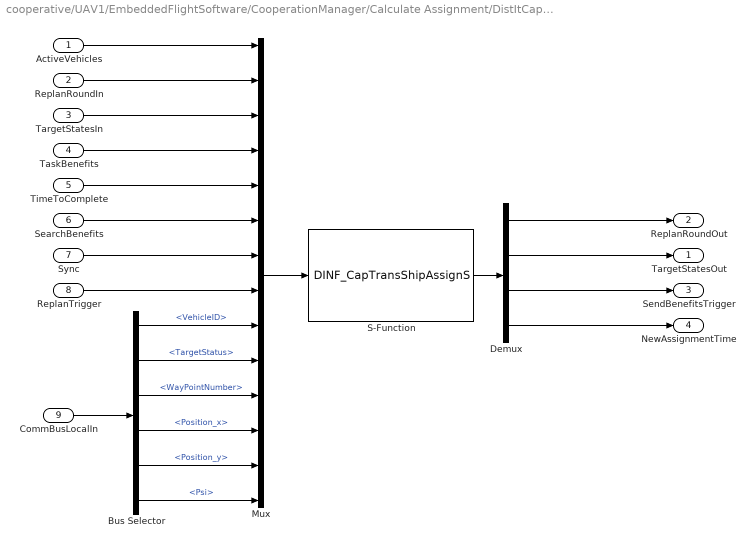
== system cooperative/UAV1/EmbeddedFlightSoftware/CooperationManager/Calculate Assignment/DistItCapTransShip/Assignment Algorithm ==
  ActiveVehicles : Inport
  ReplanRoundIn : Inport  Port=2
  TargetStatesIn : Inport  Port=3
  TaskBenefits : Inport  Port=4
  TimeToComplete : Inport  Port=5
  SearchBenefits : Inport  Port=6
  Sync : Inport  Port=7
  ReplanTrigger : Inport  Port=8
  CommBusLocalIn : Inport  Port=9
  Bus Selector : BusSelector  OutputSignals=VehicleID,EFS(com).TargetManager(com).Target Status.TargetStatus,Dynamics(com).TacticalManuevering.WayPointNumber,Dynamics(com).AC Dynamics.Position_x,Dynamics(com).AC Dynamics.Position_y,Dynamics(com).AC Dynamics.Psi
  Demux : Demux  Outputs=[2 g_MaxNumberTargets 1 1]
  Mux : Mux  Inputs=14
  S-Function : S-Function  FunctionName=DINF_CapTransShipAssignS  Parameters=g_MaxNumberTargets,g_MaxNumberVehicles  EnableBusSupport=off
  TargetStatesOut : Outport
  ReplanRoundOut : Outport  Port=2
  SendBenefitsTrigger : Outport  Port=3
  NewAssignmentTime : Outport  Port=4
  wires:
  Demux/3 -> SendBenefitsTrigger/1
  Bus Selector/6 -> Mux/14  "<Psi>"
  Bus Selector/5 -> Mux/13  "<Position_y>"
  Bus Selector/4 -> Mux/12  "<Position_x>"
  Bus Selector/3 -> Mux/11  "<WayPointNumber>"
  Bus Selector/2 -> Mux/10  "<TargetStatus>"
  Bus Selector/1 -> Mux/9  "<VehicleID>"
  CommBusLocalIn/1 -> Bus Selector/1
  Demux/1 -> ReplanRoundOut/1
  Demux/2 -> TargetStatesOut/1
  S-Function/1 -> Demux/1
  Mux/1 -> S-Function/1
  ReplanTrigger/1 -> Mux/8
  Sync/1 -> Mux/7
  SearchBenefits/1 -> Mux/6
  TimeToComplete/1 -> Mux/5
  TaskBenefits/1 -> Mux/4
  TargetStatesIn/1 -> Mux/3
  ReplanRoundIn/1 -> Mux/2
  ActiveVehicles/1 -> Mux/1
  Demux/4 -> NewAssignmentTime/1

== system cooperative/UAV1/EmbeddedFlightSoftware/CooperationManager/Calculate Assignment/DistItCapTransShip/Iteration Logic ==
  CommBusIn : Inport
  SimBusIn : Inport  Port=2
  Bus Selector : BusSelector  OutputSignals=ExternalTruth.VehicleIsDead  OutputAsBus=on
  Bus Selector1 : BusSelector  OutputSignals=TaskBenefits
  Demux : Demux  Outputs=[2,g_MaxNumberTargets,g_MaxNumberVehicles*g_MaxNumberTargets,g_MaxNumberVehicles*g_MaxNumberTargets,g_MaxNumberVehicles,1]
  Logical Operator : Logic  Operator=NOT
  Mux1 : Mux  Inputs=2
  S-Function : S-Function  FunctionName=DINF_ComparePlanS  Parameters=g_MaxNumberVehicles,g_MaxNumberTargets  EnableBusSupport=off
  ActiveVehicles : Outport
  ReplanRound : Outport  Port=2
  TargetStates : Outport  Port=3
  TaskBenefits : Outport  Port=4
  TimeToComplete : Outport  Port=5
  SearchBenefits : Outport  Port=6
  Sync : Outport  Port=7
  wires:
  Demux/6 -> Sync/1
  Demux/5 -> SearchBenefits/1
  Demux/4 -> TimeToComplete/1
  Demux/3 -> TaskBenefits/1
  Demux/2 -> TargetStates/1
  Demux/1 -> ReplanRound/1
  S-Function/1 -> Demux/1
  Mux1/1 -> S-Function/1
  Bus Selector1/1 -> Mux1/2  "<TaskBenefits>"
  CommBusIn/1 -> Bus Selector1/1
  Logical Operator/1 -> ActiveVehicles/1, Mux1/1
  SimBusIn/1 -> Bus Selector/1
  Bus Selector/1 -> Logical Operator/1

== system cooperative/UAV1/EmbeddedFlightSoftware/CooperationManager/Calculate Assignment/DistItCapTransShip/Replan Logic ==
  EnableType : Inport
  Constant : Constant
  Constant1 : Constant
  Constant2 : Constant  Value=0
  Multiport Switch : MultiPortSwitch  Inputs=4  SaturateOnIntegerOverflow=on  InputSameDT=on
  Sum : Sum  Inputs=++|  SaturateOnIntegerOverflow=on  InputSameDT=on  OutDataTypeStr=Inherit: Same as first input
  ReplanTrigger : Outport
  wires:
  Constant1/1 -> Multiport Switch/5, Multiport Switch/3
  Constant2/1 -> Multiport Switch/4, Multiport Switch/2
  Multiport Switch/1 -> ReplanTrigger/1
  Sum/1 -> Multiport Switch/1
  Constant/1 -> Sum/1
  EnableType/1 -> Sum/2

== system cooperative/UAV1/EmbeddedFlightSoftware/CooperationManager/Calculate Assignment/DistItCapTransShip/Send Benefits ==
  CommBusIn : Inport
  CommBusLocalIn : Inport  Port=2
  TargetStates : Inport  Port=3
  ReplanRound : Inport  Port=4
  Enable : EnablePort
  Bus Creator : BusCreator  Inputs=5
  Demux : Demux  Outputs=[g_MaxNumberTargets,g_MaxNumberTargets,1]
  Mux1 : Mux  Inputs=10
  S-Function : S-Function  FunctionName=DINF_CalculateBenefitsS  Parameters=g_MaxNumberTargets,g_MaxNumberVehicles  EnableBusSupport=off
  SimBusSelector : BusSelector  OutputSignals=Time,VehicleID,Dynamics(com).AC Dynamics.Position_x,Dynamics(com).AC Dynamics.Position_y,Dynamics(com).AC Dynamics.Psi,Dynamics(com).TacticalManuevering.WayPointNumber,EFS(com).TargetManager(com).SensedTargetInformation.Targets,EFS(com).SensorManager(com).ATR Combined.Desired Headings
  SimBusSelector1 : BusSelector  OutputSignals=TriggerReplan
  Algorithm Data : Outport
  wires:
  SimBusSelector1/1 -> Mux1/10  "<TriggerReplan>"
  CommBusIn/1 -> SimBusSelector1/1
  SimBusSelector/6 -> Mux1/6  "<WayPointNumber>"
  ReplanRound/1 -> Bus Creator/1  "ReplanRound"
  TargetStates/1 -> Mux1/9, Bus Creator/2  "TargetStates"
  SimBusSelector/8 -> Mux1/8  "<Desired Headings>"
  SimBusSelector/7 -> Mux1/7  "<Targets>"
  SimBusSelector/5 -> Mux1/5  "<Psi>"
  SimBusSelector/4 -> Mux1/4  "<Position_y>"
  SimBusSelector/3 -> Mux1/3  "<Position_x>"
  SimBusSelector/2 -> Mux1/2  "<VehicleID>"
  SimBusSelector/1 -> Mux1/1  "<Time>"
  CommBusLocalIn/1 -> SimBusSelector/1
  Mux1/1 -> S-Function/1
  S-Function/1 -> Demux/1
  Demux/3 -> Bus Creator/5  "SearchBenefit"
  Demux/2 -> Bus Creator/4  "TimeToComplete"
  Bus Creator/1 -> Algorithm Data/1  "Algorithm Data"
  Demux/1 -> Bus Creator/3  "TaskBenefits"

== system cooperative/UAV1/EmbeddedFlightSoftware/RouteManager/Task Status/D Latch/D Latch ==
  D : Inport
  C : EnablePort
  Q : Outport  InitialOutput=g_Tasks.Undefined
  wires:
  D/1 -> Q/1

== system cooperative/UAV1/EmbeddedFlightSoftware/RouteManager/Task Status/D Latch1/D Latch ==
  D : Inport
  C : EnablePort
  Q : Outport  InitialOutput=0
  wires:
  D/1 -> Q/1

== system cooperative/UAV1/EmbeddedFlightSoftware/RouteManager/Task Status/D Latch2/D Latch ==
  D : Inport
  C : EnablePort
  Q : Outport  InitialOutput=0
  wires:
  D/1 -> Q/1

== system cooperative/UAV1/EmbeddedFlightSoftware/RouteManager/Task Status/Task Failed Check/Task Failed Check ==
  Local (Comm) : Inport
  LastTargetState : Inport  Port=2
  Enable : EnablePort
  Bus Selector6 : BusSelector  OutputSignals=VehicleID,Dynamics(com).TacticalManuevering.AssignedTarget,Dynamics(com).TacticalManuevering.WayPointTypeCurrent,EFS(com).TargetManager(com).Target Status.TargetStatus,Dynamics(com).TacticalManuevering.WayPointNumber
  Mux1 : Mux  Inputs=7
  Save Last Task : DataStoreWrite  DataStoreName=LastWaypointType  SampleTime=g_SampleTime
  SaveLastTargetState : DataStoreWrite  DataStoreName=LastTargetState  SampleTime=g_SampleTime
  TargetStatusS : S-Function  FunctionName=TaskFailedS  Parameters=g_MaxNumberTargets  EnableBusSupport=off
  Unit Delay : UnitDelay  SampleTime=g_SampleTime
  Unit Delay1 : UnitDelay  SampleTime=g_SampleTime
  TaskFailed : Outport
  wires:
  Bus Selector6/5 -> Mux1/7  "<WayPointNumber>"
  LastTargetState/1 -> Mux1/6
  Bus Selector6/4 -> Mux1/5, SaveLastTargetState/1  "<TargetStatus>"
  Unit Delay1/1 -> Mux1/3
  Bus Selector6/1 -> Mux1/1  "<VehicleID>"
  Unit Delay/1 -> Mux1/2
  TargetStatusS/1 -> TaskFailed/1
  Mux1/1 -> TargetStatusS/1
  Bus Selector6/2 -> Unit Delay/1  "<AssignedTarget>"
  Local (Comm)/1 -> Bus Selector6/1
  Bus Selector6/3 -> Mux1/4, Unit Delay1/1, Save Last Task/1  "<WayPointTypeCurrent>"

== system cooperative/UAV1/EmbeddedFlightSoftware/SensorManager/ATR Single/SingleATR/Assume Responsibility ==
  NewTargets : Inport
  VehicleID : Inport  Port=2
  Enable : EnablePort
  Mux : Mux  Inputs=2
  S-Function : S-Function  FunctionName=DAINF_AssumeDutyS  EnableBusSupport=off
  wires:
  NewTargets/1 -> Mux/2
  VehicleID/1 -> Mux/1
  Mux/1 -> S-Function/1

== system cooperative/UAV1/EmbeddedFlightSoftware/CooperationManager/Calculate Assignment/DistAuctItCapTransShip/Assignment Algorithm/Auction Algorithm ==
  VehicleID : Inport
  Enable : EnablePort  StatesWhenEnabling=reset
  Auction Algorithm : S-Function  FunctionName=DAINF_AuctionS  EnableBusSupport=off
  AuctionData : Outport
  wires:
  VehicleID/1 -> Auction Algorithm/1
  Auction Algorithm/1 -> AuctionData/1

== system cooperative/UAV1/EmbeddedFlightSoftware/CooperationManager/Calculate Assignment/DistAuctItCapTransShip/Assignment Algorithm/Iteration Algorithm ==
  RoundComplete : Inport
  ReplanTrigger : Inport  Port=2
  CommBusLocalIn : Inport  Port=3
  Enable : EnablePort  StatesWhenEnabling=reset
  Bus Selector : BusSelector  OutputSignals=VehicleID,EFS(com).TargetManager(com).Target Status.TargetStatus,Dynamics(com).TacticalManuevering.WayPointNumber,Dynamics(com).AC Dynamics.Position_x,Dynamics(com).AC Dynamics.Position_y,Dynamics(com).AC Dynamics.Psi
  Demux : Demux  Outputs=[g_MaxNumberTargets,1,1,1]
  Iteration Algorithm : S-Function  FunctionName=DAINF_IterationControlS  EnableBusSupport=off
  Mux : Mux  Inputs=8
  StoreBenefits : Outport  OutputWhenDisabled=reset  InitialOutput=[0]
  TargetStates : Outport  Port=2
  AssignmentCompelte : Outport  Port=3  OutputWhenDisabled=reset  InitialOutput=[0]
  NewAssignmentTime : Outport  Port=4  OutputWhenDisabled=reset  InitialOutput=[0]
  wires:
  Demux/3 -> AssignmentCompelte/1
  Bus Selector/6 -> Mux/8  "<Psi>"
  Bus Selector/5 -> Mux/7  "<Position_y>"
  Bus Selector/4 -> Mux/6  "<Position_x>"
  Bus Selector/3 -> Mux/5  "<WayPointNumber>"
  Bus Selector/2 -> Mux/4  "<TargetStatus>"
  Bus Selector/1 -> Mux/3  "<VehicleID>"
  Demux/2 -> StoreBenefits/1
  CommBusLocalIn/1 -> Bus Selector/1
  Mux/1 -> Iteration Algorithm/1
  ReplanTrigger/1 -> Mux/2
  RoundComplete/1 -> Mux/1
  Demux/1 -> TargetStates/1
  Iteration Algorithm/1 -> Demux/1
  Demux/4 -> NewAssignmentTime/1
